simulink model "ur5_simulink_ros2_ibvs_mpc_old"  (R2023b)
settings: Solver=FixedStepAuto  StartTime=0.0  StopTime=inf  RelTol=1e-3
model workspace (MAT data in the model file):
  SL_ROS_VariableLengthArrays_MaxSizes.CommonInfo.ArrayTruncateAction = 'EmitWarning'
  SL_ROS_VariableLengthArrays_MaxSizes.MsgTypeMap = containers.Map
  SL_ROS_VariableLengthArrays_MaxSizes.MsgTypeMap.serialization.keys = {'example_interfaces/Float64MultiArray'}
  SL_ROS_VariableLengthArrays_MaxSizes.MsgTypeMap.serialization.values{1}.PropertyName = 'data'
  SL_ROS_VariableLengthArrays_MaxSizes.MsgTypeMap.serialization.values{1}.DataType = 'double'
  SL_ROS_VariableLengthArrays_MaxSizes.MsgTypeMap.serialization.values{1}.MaxLength = 1
  SL_ROS_VariableLengthArrays_MaxSizes.MsgTypeMap.serialization.uniformity = 0
  SL_ROS_VariableLengthArrays_MaxSizes.MsgTypeMap.serialization.keyType = 'char'
  SL_ROS_VariableLengthArrays_MaxSizes.MsgTypeMap.serialization.valueType = 'any'
undefined symbols (not defined in the file or in its folder): data, data_SL_Info
libraries: ros2lib x12, robotmaniplib x3, robotcorelib x2, mpclib x1, spsFirstOrderFilterLib x1
settings Model: SimulationMode=accelerator  Creator=81232  LastModifiedBy=ias-lab-701
settings OptimizationCC: EnhancedBackFolding=on  PassReuseOutputArgsAs=Individual arguments  ZeroExternalMemoryAtStartup=off  ZeroInternalMemoryAtStartup=off  MaxStackSize=64  OptimizeBlockOrder=speed  DifferentSizesBufferReuse=on  OptimizationCustomize=off  EfficientTunableParamExpr=on
settings DebuggingCC: ParameterTunabilityLossMsg=error
settings ModelReferenceCC: EnableRefExpFcnMdlSchedulingChecks=on
settings SFSimCC: MATLABDynamicMemAlloc=off
settings RTWCC: Description=Embedded Coder  SystemTargetFile=ert.tlc  HardwareBoard=Robot Operating System 2 (ROS 2)  TLCOptions="-aInlineSetEventsForThisBaseRateFcn=TLC_FALSE -aSuppressMultiTaskScheduler=TLC_FALSE  -aRateBasedStepFcn=0"  TemplateMakefile=ert_default_tmf  Toolchain=Colcon Tools  TargetLang=C++
settings CodeAppCC: ForceParamTrailComments=on  IgnoreCustomStorageClasses=off  OperatorAnnotations=on  SimulinkDataObjDesc=on  SFDataObjDesc=on  InsertBlockDesc=on
settings ERTTargetCC: CodeInterfacePackaging=C++ class  RootIOFormat=Structure reference

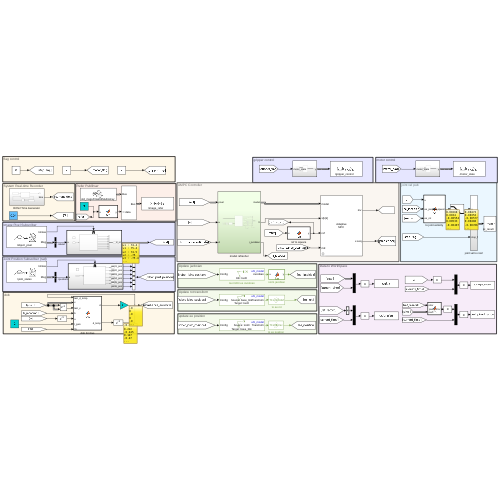
[thumbnail: Simulink's stored preview of the top-level diagram]
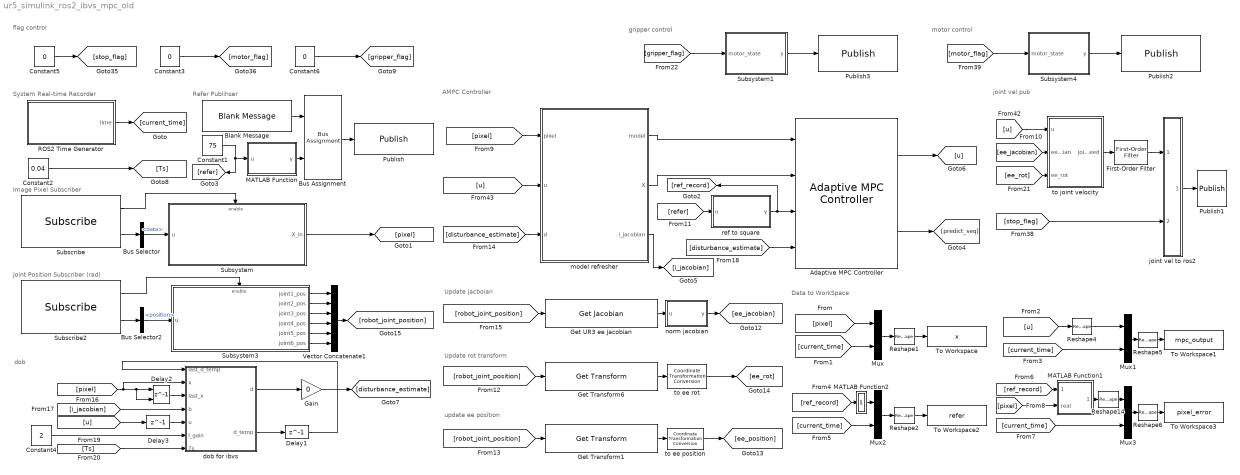
== system ur5_simulink_ros2_ibvs_mpc_old ==
  note: dob
  note: joint vel pub
  note: update ee position
  note: Update rot transform
  note: Joint Position Subscriber (rad)
  note: Refer Publihser
  note: Data to WorkSpace
  note: System Real-time Recorder
  note: Image Pixel Subscriber
  note: AMPC Controller
  note: Update jacboian
  note: flag control
  note: motor control
  note: gripper control
  Adaptive MPC Controller : mpclib/Adaptive MPC Controller  SCDEnableBlockLinearizationSpecification=on  mpcobj=mpcobj  enable_value=0  updateMPCinCallerWorkspace=on  md_inport=on  mv_inport=off  uref_inport=off  return_cost=off  return_mvseq=off  return_qpstatus=off  return_xseq=on  return_state=off  return_ovseq=off  state_inport=on  isltv_plant=off  umin_inport=off  umax_inport=off  ymin_inport=off  ymax_inport=off  cc_inport=off  ywt_inport=off  uwt_inport=off  duwt_inport=off  rhoeps_inport=off  pm_inport=off  MaximumP=10  HorizonChoice=FixedHorizon  BlockDataType=double  SampleTimeInherited=off  switch_inport=off
  Blank Message : ros2lib/Blank Message  messageClass=Message  entityType=std_msgs/Float64MultiArray  messageType=std_msgs/Float64MultiArray  SampleTime=inf
      settings: LibrarySourceBlock=roslib/ROS 2/Blank Message
  Bus Assignment : BusAssignment  AssignedSignals=data
  Bus Selector : BusSelector  OutputSignals=data
  Bus Selector2 : BusSelector  OutputSignals=position
  Constant1 : Constant  Value=75
  Constant2 : Constant  Value=0.04
  Constant3 : Constant  Value=0
  Constant4 : Constant  Value=2
  Constant5 : Constant  Value=0
  Constant6 : Constant  Value=0
  Delay1 : Delay  DelayLength=1
  Delay2 : Delay  DelayLength=1  InitialConditionSource=Input port
      settings: InputPortMap=u0,p4
  Delay3 : Delay  DelayLength=1
  First-Order Filter : spsFirstOrderFilterLib/First-Order Filter  FilterType=Lowpass  Tc=10e-2  Ts=0  Initialize=off  Vac_Init=[0, 0, 60]  Vdc_Init=0  PlotResponse=off  FreqRange="[0,  200,  1]"
  Gain : Gain  Gain=0
  Get Transform1 : robotmaniplib/Get Transform  RigidBodyTree=ur5_model  SourceBody=tool0  TargetBody=base_link  SimulateUsing=Interpreted execution
  Get Transform6 : robotmaniplib/Get Transform  RigidBodyTree=ur5_model  SourceBody=base_link  TargetBody=tool0  SimulateUsing=Interpreted execution
  Get UR3 ee Jacobian : robotmaniplib/Get Jacobian  RigidBodyTree=ur5_model  EndEffector=tool0  SimulateUsing=Interpreted execution
  MATLAB Function : MATLAB Function  TreatAsAtomicUnit=on
  MATLAB Function1 : MATLAB Function  TreatAsAtomicUnit=on
  MATLAB Function2 : MATLAB Function  TreatAsAtomicUnit=on
  Mux{,1..3} (4 alike) : Mux  Inputs=2
  Publish : ros2lib/Publish  topicSource=Specify your own  topic=/image_refer  messageType=std_msgs/Float64MultiArray  QOSHistory=Keep last  QOSDepth=1  QOSReliability=Reliable  QOSDurability=Volatile
      settings: LibrarySourceBlock=roslib/ROS 2/Publish
  Publish1 : ros2lib/Publish  topicSource=Select from ROS network  topic=/simulink_mpc_result  messageType=std_msgs/Float64MultiArray  QOSHistory=Keep last  QOSDepth=1  QOSReliability=Reliable  QOSDurability=Volatile
      settings: LibrarySourceBlock=roslib/ROS 2/Publish
  Publish2 : ros2lib/Publish  topicSource=Select from ROS network  topic=/motor_state  messageType=std_msgs/Int64  QOSHistory=Keep last  QOSDepth=1  QOSReliability=Reliable  QOSDurability=Volatile
      settings: LibrarySourceBlock=roslib/ROS 2/Publish
  Publish3 : ros2lib/Publish  topicSource=Select from ROS network  topic=/gripper_control  messageType=std_msgs/Int64  QOSHistory=Keep last  QOSDepth=1  QOSReliability=Reliable  QOSDurability=Volatile
      settings: LibrarySourceBlock=roslib/ROS 2/Publish
  ROS2 Time Generator : Subsystem
  Reshape1 : Reshape  OutputDimensionality=Customize  OutputDimensions=[9]
  Reshape14 : Reshape  OutputDimensionality=Customize  OutputDimensions=[8,1]
  Reshape2 : Reshape  OutputDimensionality=Customize  OutputDimensions=[9]
  Reshape4 : Reshape  OutputDimensionality=Customize  OutputDimensions=[6,1]
  Reshape5 : Reshape  OutputDimensionality=Customize  OutputDimensions=[7]
  Reshape6 : Reshape  OutputDimensionality=Customize  OutputDimensions=[9]
  Subscribe : ros2lib/Subscribe  topicSource=Select from ROS network  topic=/object_pixel  messageType=std_msgs/Float64MultiArray  sampleTime=-1  QOSHistory=Keep last  QOSDepth=1  QOSReliability=Reliable  QOSDurability=Volatile
  Subscribe2 : ros2lib/Subscribe  topicSource=Select from ROS network  topic=/joint_states  messageType=sensor_msgs/JointState  sampleTime=-1  QOSHistory=Keep last  QOSDepth=1  QOSReliability=Reliable  QOSDurability=Volatile
  Subsystem : Subsystem
  Subsystem1 : Subsystem
  Subsystem3 : Subsystem
  Subsystem4 : Subsystem
  To Workspace : ToWorkspace  VariableName=x  SaveFormat=Timeseries  SampleTime=-1
  To Workspace1 : ToWorkspace  VariableName=mpc_output  SaveFormat=Timeseries  SampleTime=-1
  To Workspace2 : ToWorkspace  VariableName=refer  SaveFormat=Timeseries  SampleTime=-1
  To Workspace3 : ToWorkspace  VariableName=pixel_error  SaveFormat=Timeseries  SampleTime=-1
  Vector Concatenate1 : Concatenate  NumInputs=6
  dob for ibvs : MATLAB Function  TreatAsAtomicUnit=on
  joint vel to ros2 : Subsystem
  model refresher : Subsystem
  norm jacobian : MATLAB Function  TreatAsAtomicUnit=on
  ref to square : MATLAB Function  TreatAsAtomicUnit=on
  to ee position : robotcorelib/Coordinate Transformation Conversion  InputRepresentation=Homogeneous Transformation  InputEulerSequence=ZYX  ShowTrVecInputPort=on  OutputRepresentation=Translation Vector  OutputEulerSequence=ZYX  ShowTrVecOutputPort=off  SimulateUsing=Interpreted execution
  to ee rot : robotcorelib/Coordinate Transformation Conversion  InputRepresentation=Homogeneous Transformation  InputEulerSequence=ZYX  ShowTrVecInputPort=on  OutputRepresentation=Rotation Matrix  OutputEulerSequence=ZYX  ShowTrVecOutputPort=off  SimulateUsing=Interpreted execution
  to joint velocity : MATLAB Function  TreatAsAtomicUnit=on
  wires:
  Bus Selector/1 -> Subsystem/1(u)  "<data>"
  Subscribe/2 -> Bus Selector/1
  Subscribe/1 -> Subsystem/Enable
  ROS2 Time Generator/1(time) -> [current_time]
  Subsystem/1(X_in) -> [pixel]
  [pixel] -> Mux/1
  [current_time] -> Mux/2
  [u] -> Reshape4/1
  [current_time] -> Mux1/2
  Blank Message/1 -> Bus Assignment/1
  Bus Assignment/1 -> Publish/1
  Constant1/1 -> [refer], MATLAB Function/1(u)
  MATLAB Function/1(y) -> Bus Assignment/2
  [current_time] -> Mux2/2
  Mux2/1 -> Reshape2/1
  [current_time] -> Mux3/2
  [ref_record] -> MATLAB Function1/1(refer)
  [pixel] -> MATLAB Function1/2(real)
  ref to square/1(y) -> [ref_record], Adaptive MPC Controller/3
  [refer] -> ref to square/1(u)
  [disturbance_estimate] -> Adaptive MPC Controller/4
  joint vel to ros2/1(Out1) -> Publish1/1
  Adaptive MPC Controller/2 -> [predict_seq]
  Mux3/1 -> Reshape6/1
  MATLAB Function1/1(pixel_error) -> Reshape14/1
  Reshape14/1 -> Mux3/1
  Reshape4/1 -> Mux1/1
  Mux1/1 -> Reshape5/1
  Reshape5/1 -> To Workspace1/1
  Reshape6/1 -> To Workspace3/1
  Subscribe2/2 -> Bus Selector2/1
  Bus Selector2/1 -> Subsystem3/1(u)  "<position>"
  Subscribe2/1 -> Subsystem3/Enable
  model refresher/1(model) -> Adaptive MPC Controller/1
  model refresher/2(X) -> Adaptive MPC Controller/2
  Subsystem3/1(joint1_pos) -> Vector Concatenate1/1
  Subsystem3/2(joint2_pos) -> Vector Concatenate1/2
  Subsystem3/3(joint3_pos) -> Vector Concatenate1/3
  Subsystem3/4(joint4_pos) -> Vector Concatenate1/4
  Subsystem3/5(joint5_pos) -> Vector Concatenate1/5
  Subsystem3/6(joint6_pos) -> Vector Concatenate1/6
  norm jacobian/1(y) -> [ee_jacobian]
  Get UR3 ee Jacobian/1 -> norm jacobian/1(u)
  [pixel] -> model refresher/1(pixel)
  [robot_joint_position] -> Get Transform6/1
  Get Transform6/1 -> to ee rot/1
  to ee rot/1 -> [ee_rot]
  to ee position/1 -> [ee_position]
  Get Transform1/1 -> to ee position/1
  [robot_joint_position] -> Get UR3 ee Jacobian/1
  [robot_joint_position] -> Get Transform1/1
  Vector Concatenate1/1 -> [robot_joint_position]
  [u] -> model refresher/2(u)
  [disturbance_estimate] -> model refresher/3(d)
  Mux/1 -> Reshape1/1
  Reshape1/1 -> To Workspace/1
  Reshape2/1 -> To Workspace2/1
  Delay1/1 -> dob for ibvs/1(last_d_temp)
  [u] -> Delay3/1
  dob for ibvs/2(d_temp) -> Delay1/1
  [i_jacobian] -> dob for ibvs/4(b)
  Constant4/1 -> dob for ibvs/6(l_gain)
  [pixel] -> Delay2/2, Delay2/1, dob for ibvs/2(x)
  Delay2/1 -> dob for ibvs/3(last_x)
  Delay3/1 -> dob for ibvs/5(u)
  Gain/1 -> [disturbance_estimate]
  MATLAB Function2/1(y) -> Mux2/1
  [ref_record] -> MATLAB Function2/1(u)
  dob for ibvs/1(d) -> Gain/1
  [Ts] -> dob for ibvs/7(Ts)
  Constant2/1 -> [Ts]
  Constant5/1 -> [stop_flag]
  Constant3/1 -> [motor_flag]
  [motor_flag] -> Subsystem4/1(motor_state)
  Subsystem4/1(y) -> Publish2/1
  [stop_flag] -> joint vel to ros2/2(stop_flag)
  Constant6/1 -> [gripper_flag]
  Subsystem1/1(y) -> Publish3/1
  [gripper_flag] -> Subsystem1/1(motor_state)
  [u] -> to joint velocity/1(u)
  [ee_jacobian] -> to joint velocity/2(ee_jacobian)
  [ee_rot] -> to joint velocity/3(ee_rot)
  Adaptive MPC Controller/1 -> [u]
  to joint velocity/1(joint_speed) -> First-Order Filter/1
  First-Order Filter/1 -> joint vel to ros2/1(u)
  model refresher/3(i_jacobian) -> [i_jacobian]

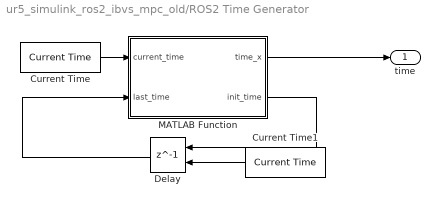
== system ur5_simulink_ros2_ibvs_mpc_old/ROS2 Time Generator ==
  Current Time : ros2lib/Current Time  OutputFormat=double  SampleTime=-1  ModelName=ur5_simulink_ros2_ibvs_mpc_old
      settings: LibrarySourceBlock=roslib/ROS 2/Current Time
  Current Time1 : ros2lib/Current Time  OutputFormat=double  SampleTime=-1  ModelName=ur5_simulink_ros2_ibvs_mpc_old
      settings: LibrarySourceBlock=roslib/ROS 2/Current Time
  Delay : Delay  DelayLength=1  InitialConditionSource=Input port
      settings: InputPortMap=u0,p4
  MATLAB Function : MATLAB Function  TreatAsAtomicUnit=on
  time : Outport
  wires:
  Delay/1 -> MATLAB Function/2(last_time)
  Current Time1/1 -> Delay/2
  MATLAB Function/2(init_time) -> Delay/1
  Current Time/1 -> MATLAB Function/1(current_time)
  MATLAB Function/1(time_x) -> time/1

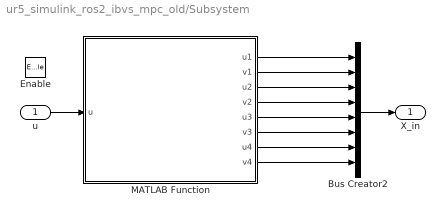
== system ur5_simulink_ros2_ibvs_mpc_old/Subsystem ==
  u : Inport
  Enable : EnablePort
  Bus Creator2 : BusCreator  Inputs=8
  MATLAB Function : MATLAB Function  TreatAsAtomicUnit=on
  X_in : Outport
  wires:
  MATLAB Function/2(v1) -> Bus Creator2/2
  MATLAB Function/5(u3) -> Bus Creator2/5
  MATLAB Function/1(u1) -> Bus Creator2/1
  MATLAB Function/4(v2) -> Bus Creator2/4
  MATLAB Function/3(u2) -> Bus Creator2/3
  u/1 -> MATLAB Function/1(u)
  Bus Creator2/1 -> X_in/1
  MATLAB Function/6(v3) -> Bus Creator2/6
  MATLAB Function/7(u4) -> Bus Creator2/7
  MATLAB Function/8(v4) -> Bus Creator2/8

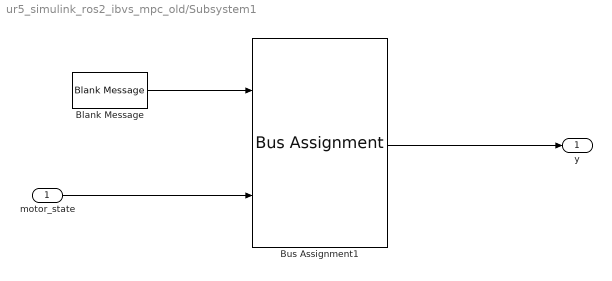
== system ur5_simulink_ros2_ibvs_mpc_old/Subsystem1 ==
  motor_state : Inport
  Blank Message : ros2lib/Blank Message  messageClass=Message  entityType=std_msgs/Int64  messageType=std_msgs/Int64  SampleTime=inf
  Bus Assignment1 : BusAssignment  AssignedSignals=data
  y : Outport
  wires:
  Blank Message/1 -> Bus Assignment1/1
  Bus Assignment1/1 -> y/1
  motor_state/1 -> Bus Assignment1/2

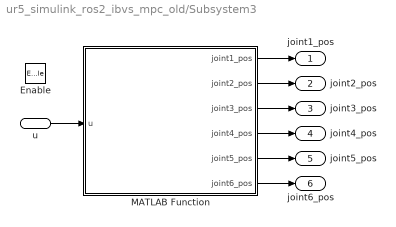
== system ur5_simulink_ros2_ibvs_mpc_old/Subsystem3 ==
  u : Inport
  Enable : EnablePort
  MATLAB Function : MATLAB Function  TreatAsAtomicUnit=on
  joint1_pos : Outport
  joint2_pos : Outport  Port=2
  joint3_pos : Outport  Port=3
  joint4_pos : Outport  Port=4
  joint5_pos : Outport  Port=5
  joint6_pos : Outport  Port=6
  wires:
  u/1 -> MATLAB Function/1(u)
  MATLAB Function/1(joint1_pos) -> joint1_pos/1
  MATLAB Function/2(joint2_pos) -> joint2_pos/1
  MATLAB Function/3(joint3_pos) -> joint3_pos/1
  MATLAB Function/4(joint4_pos) -> joint4_pos/1
  MATLAB Function/5(joint5_pos) -> joint5_pos/1
  MATLAB Function/6(joint6_pos) -> joint6_pos/1

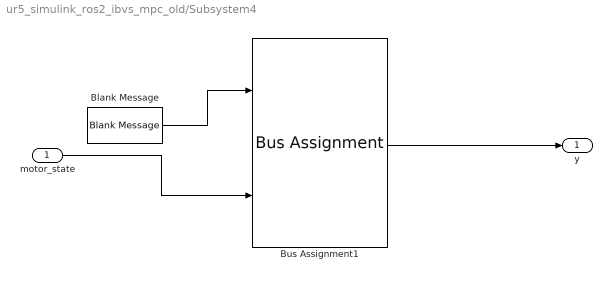
== system ur5_simulink_ros2_ibvs_mpc_old/Subsystem4 ==
  motor_state : Inport
  Blank Message : ros2lib/Blank Message  messageClass=Message  entityType=std_msgs/Int64  messageType=std_msgs/Int64  SampleTime=inf
  Bus Assignment1 : BusAssignment  AssignedSignals=data
  y : Outport
  wires:
  Blank Message/1 -> Bus Assignment1/1
  Bus Assignment1/1 -> y/1
  motor_state/1 -> Bus Assignment1/2

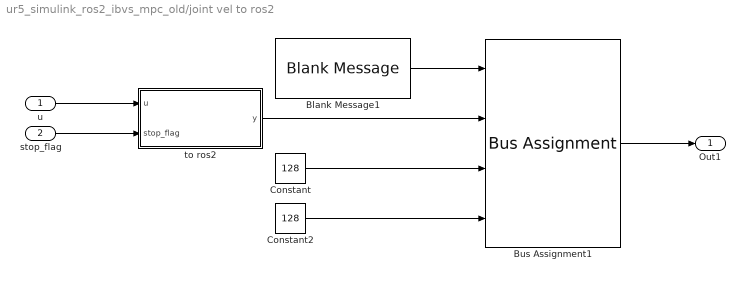
== system ur5_simulink_ros2_ibvs_mpc_old/joint vel to ros2 ==
  u : Inport
  stop_flag : Inport  Port=2
  Blank Message1 : ros2lib/Blank Message  messageClass=Message  entityType=std_msgs/Float64MultiArray  messageType=std_msgs/Float64MultiArray  SampleTime=inf
      settings: LibrarySourceBlock=roslib/ROS 2/Blank Message
  Bus Assignment1 : BusAssignment  AssignedSignals=data,data_SL_Info.CurrentLength,data_SL_Info.ReceivedLength
  Constant : Constant  Value=128  OutDataTypeStr=uint32
  Constant2 : Constant  Value=128  OutDataTypeStr=uint32
  to ros2 : MATLAB Function  TreatAsAtomicUnit=on
  Out1 : Outport
  wires:
  u/1 -> to ros2/1(u)
  to ros2/1(y) -> Bus Assignment1/2
  Constant2/1 -> Bus Assignment1/4
  Constant/1 -> Bus Assignment1/3
  Blank Message1/1 -> Bus Assignment1/1
  Bus Assignment1/1 -> Out1/1
  stop_flag/1 -> to ros2/2(stop_flag)

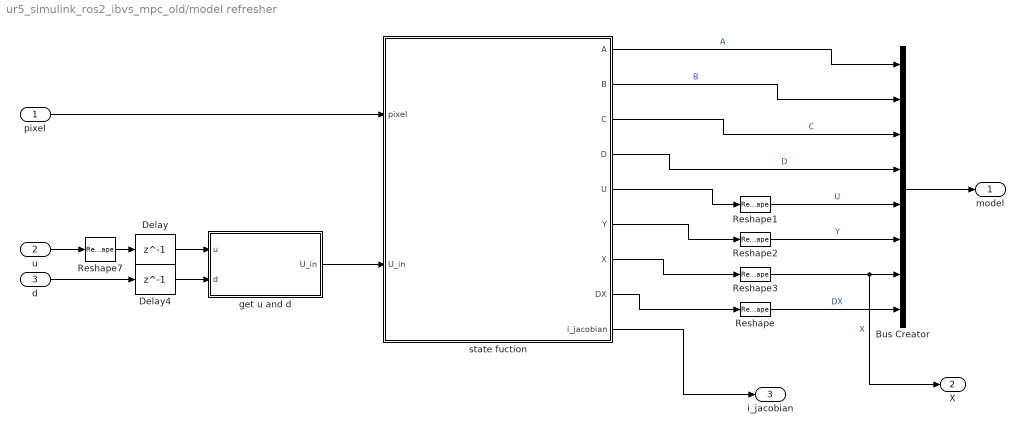
== system ur5_simulink_ros2_ibvs_mpc_old/model refresher ==
  pixel : Inport
  u : Inport  Port=2
  d : Inport  Port=3
  Bus Creator : BusCreator  Inputs=8
  Delay : Delay  DelayLength=1
  Delay4 : Delay  DelayLength=1
  Reshape : Reshape  OutputDimensionality=Customize  OutputDimensions=[8,1]
  Reshape1 : Reshape  OutputDimensionality=Customize  OutputDimensions=[14,1]
  Reshape2 : Reshape  OutputDimensionality=Customize  OutputDimensions=[8,1]
  Reshape3 : Reshape  OutputDimensionality=Customize  OutputDimensions=[8,1]
  Reshape7 : Reshape  OutputDimensionality=Customize  OutputDimensions=[6]
  get u and d : Subsystem
  state fuction : MATLAB Function  TreatAsAtomicUnit=on
  model : Outport
  X : Outport  Port=2
  i_jacobian : Outport  Port=3
  wires:
  state fuction/2(B) -> Bus Creator/2  "B"
  state fuction/5(U) -> Reshape1/1
  pixel/1 -> state fuction/1(pixel)
  state fuction/1(A) -> Bus Creator/1  "A"
  state fuction/4(D) -> Bus Creator/4  "D"
  state fuction/3(C) -> Bus Creator/3  "C"
  get u and d/1(U_in) -> state fuction/2(U_in)
  state fuction/6(Y) -> Reshape2/1
  state fuction/7(X) -> Reshape3/1
  state fuction/8(DX) -> Reshape/1
  Reshape1/1 -> Bus Creator/5  "U"
  Reshape2/1 -> Bus Creator/6  "Y"
  Reshape3/1 -> Bus Creator/7, X/1  "X"
  Reshape/1 -> Bus Creator/8  "DX"
  Bus Creator/1 -> model/1
  Reshape7/1 -> Delay/1
  Delay4/1 -> get u and d/2(d)
  Delay/1 -> get u and d/1(u)
  u/1 -> Reshape7/1
  d/1 -> Delay4/1
  state fuction/9(i_jacobian) -> i_jacobian/1

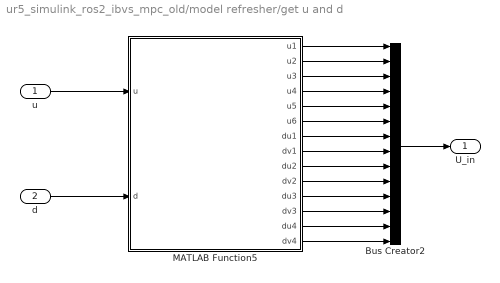
== system ur5_simulink_ros2_ibvs_mpc_old/model refresher/get u and d ==
  u : Inport
  d : Inport  Port=2
  Bus Creator2 : BusCreator  Inputs=14
  MATLAB Function5 : MATLAB Function  TreatAsAtomicUnit=on
  U_in : Outport
  wires:
  MATLAB Function5/3(u3) -> Bus Creator2/3
  MATLAB Function5/1(u1) -> Bus Creator2/1
  MATLAB Function5/11(du3) -> Bus Creator2/11
  MATLAB Function5/8(dv1) -> Bus Creator2/8
  MATLAB Function5/12(dv3) -> Bus Creator2/12
  MATLAB Function5/9(du2) -> Bus Creator2/9
  MATLAB Function5/13(du4) -> Bus Creator2/13
  MATLAB Function5/14(dv4) -> Bus Creator2/14
  MATLAB Function5/6(u6) -> Bus Creator2/6
  MATLAB Function5/4(u4) -> Bus Creator2/4
  MATLAB Function5/5(u5) -> Bus Creator2/5
  MATLAB Function5/7(du1) -> Bus Creator2/7
  MATLAB Function5/2(u2) -> Bus Creator2/2
  MATLAB Function5/10(dv2) -> Bus Creator2/10
  u/1 -> MATLAB Function5/1(u)
  Bus Creator2/1 -> U_in/1
  d/1 -> MATLAB Function5/2(d)

== matlab function ur5_simulink_ros2_ibvs_mpc_old/joint vel to ros2/to ros2 ==
  data: u input; y output; stop_flag input
function y  = fcn(u, stop_flag)
    y = zeros(128,1);
    if stop_flag==1
        y(1) = 0;
        y(2) = 0;
        y(3) = 0;
        y(4) = 0;
        y(5) = 0;
        y(6) = 0;
    else
        y(1) = u(1);
        y(2) = u(2);
        y(3) = u(3);
        y(4) = u(4);
        y(5) = u(5);
        y(6) = u(6);
    end
end

== matlab function ur5_simulink_ros2_ibvs_mpc_old/MATLAB Function2 ==
  data: u input; y output
function y = fcn(u)
y = u(1:8);

== matlab function ur5_simulink_ros2_ibvs_mpc_old/model refresher/get u and d/MATLAB Function5 ==
  data: u input; u1 output; u2 output; u3 output; u4 output; u5 output; u6 output; du1 output; dv1 output; du2 output; dv2 output; du3 output; dv3 output; du4 output; dv4 output; d input
function [u1,u2,u3,u4,u5,u6,du1,dv1,du2,dv2,du3,dv3,du4,dv4] = fcn(u,d)
u1 = u(1);
u2 = u(2);
u3 = u(3);
u4 = u(4);
u5 = u(5);
u6 = u(6);
%disturbance
du1 = d(1);
dv1 = d(2);
du2 = d(3);
dv2 = d(4);
du3 = d(5);
dv3 = d(6);
du4 = d(7);
dv4 = d(8);

== matlab function ur5_simulink_ros2_ibvs_mpc_old/to joint velocity ==
  data: u input; joint_speed output; ee_jacobian input; ee_rot input
function joint_speed  = fcn(u, ee_jacobian, ee_rot)
    rot_mat = [ee_rot,zeros(3,3);zeros(3,3),ee_rot];
    new_jacobian = rot_mat*ee_jacobian;
    joint_speed = new_jacobian\u;
end

== matlab function ur5_simulink_ros2_ibvs_mpc_old/norm jacobian ==
  data: u input; y output size=[6,6]
function y = fcn(u)
firstThreeColumns =u(1:3, :);
lastThreeColumns = u(4:6, :);
y = [lastThreeColumns;firstThreeColumns];

== matlab function ur5_simulink_ros2_ibvs_mpc_old/Subsystem3/MATLAB Function ==
  data: u input; joint1_pos output; joint2_pos output; joint3_pos output; joint4_pos output; joint5_pos output; joint6_pos output
function [joint1_pos,joint2_pos,joint3_pos,joint4_pos,joint5_pos,joint6_pos] = fcn(u)
joint1_pos = u(6);
joint2_pos = u(1);
joint3_pos = u(2);
joint4_pos = u(3);
joint5_pos = u(4);
joint6_pos = u(5);

== matlab function ur5_simulink_ros2_ibvs_mpc_old/Subsystem/MATLAB Function ==
  data: u input; u1 output; v1 output; u2 output; v2 output; u3 output; v3 output; u4 output; v4 output
function [u1,v1,u2,v2,u3,v3,u4,v4] = fcn(u)
u_center = 320;
v_center = 240;
u1 = u(1) - u_center;
v1 = u(2) - v_center;
u2 = u(3) - u_center;
v2 = u(4) - v_center;
u3 = u(5) - u_center;
v3 = u(6) - v_center;
u4 = u(7) - u_center;
v4 = u(8) - v_center;

== matlab function ur5_simulink_ros2_ibvs_mpc_old/ROS2 Time Generator/MATLAB Function ==
  data: current_time input; last_time input; time_x output; init_time output
function [time_x,init_time] = fcn(current_time, last_time)
init_time = last_time;
time_x = current_time-last_time;

== matlab function ur5_simulink_ros2_ibvs_mpc_old/dob for ibvs ==
  data: last_d_temp input size=8; x input size=8; last_x input size=8; b input size=[8,6]; u input size=6; d output size=8; l_gain input; d_temp output size=8; Ts input
function [d,d_temp] = fcn(last_d_temp,x,last_x,b,u,l_gain,Ts)
d_temp = last_d_temp - Ts*l_gain*last_d_temp + l_gain*(x-last_x-Ts*b*u);
d = d_temp;

== matlab function ur5_simulink_ros2_ibvs_mpc_old/MATLAB Function ==
  data: u input; y output
function y = fcn(u)
y = zeros(1,128);
y(1) = u;
y(2) = u;
y(3) = u;
y(4) = -u;
y(5) = -u;
y(6) = -u;
y(7) = -u;
y(8) = u;

== matlab function ur5_simulink_ros2_ibvs_mpc_old/MATLAB Function1 ==
  data: refer input; pixel_error output; real input
function pixel_error = fcn(refer,real)
pixel_error = zeros(8,1);
pixel_error(1) = refer(1) -real(1);
pixel_error(2) = refer(2) -real(2);
pixel_error(3) = refer(3) -real(3);
pixel_error(4) = refer(4) -real(4);
pixel_error(5) = refer(5) -real(5);
pixel_error(6) = refer(6) -real(6);
pixel_error(7) = refer(7) -real(7);
pixel_error(8) = refer(8) -real(8);

== matlab function ur5_simulink_ros2_ibvs_mpc_old/model refresher/state fuction ==
  data: pixel input; A output; U_in input; B output; C output; D output; U output; Y output; X output; DX output; i_jacobian output
function [A, B, C, D, U, Y, X, DX,i_jacobian] = fcn(pixel, U_in)
A = zeros(8,8);
C = eye(8);
D = zeros(8,14);
X= pixel;
[B,i_jacobian] = getContinuous(X);
U=U_in;
DZ = B*U_in;
DX = [DZ(1);DZ(2);DZ(3);DZ(4);DZ(5);DZ(6);DZ(7);DZ(8)];
Y=X;

function  [b_,i_jacobian_] = getContinuous(x_)
b_ = zeros(8, 14);
% states
u_1 = x_(1);
v_1 = x_(2);
u_2 = x_(3);
v_2 = x_(4);
u_3 = x_(5);
v_3 = x_(6);
u_4 = x_(7);
v_4 = x_(8);
% parameters
f = 900;            %focal length of realsenseD455=1930um
p_size = 0;        %Pixel Size of realsenseD4455=3um
f_pixel = 633;       %the focal length in pixels f/p_size
Z = 0.25;             %Depth estimate for four points
% image jcobian
i_jacobian_ = [-f_pixel/Z,0,u_1/Z,u_1*v_1/f_pixel,-(f_pixel^2+u_1^2)/f_pixel,v_1;
             0,-f_pixel/Z,v_1/Z,(f_pixel^2+v_1^2)/f_pixel,-u_1*v_1/f_pixel,-u_1;
             -f_pixel/Z,0,u_2/Z,u_2*v_2/f_pixel,-(f_pixel^2+u_2^2)/f_pixel,v_2;
             0,-f_pixel/Z,v_2/Z,(f_pixel^2+v_2^2)/f_pixel,-u_2*v_2/f_pixel,-u_2;
             -f_pixel/Z,0,u_3/Z,u_3*v_3/f_pixel,-(f_pixel^2+u_3^2)/f_pixel,v_3;
             0,-f_pixel/Z,v_3/Z,(f_pixel^2+v_3^2)/f_pixel,-u_3*v_3/f_pixel,-u_3;
             -f_pixel/Z,0,u_4/Z,u_4*v_4/f_pixel,-(f_pixel^2+u_4^2)/f_pixel,v_4;
             0,-f_pixel/Z,v_4/Z,(f_pixel^2+v_4^2)/f_pixel,-u_4*v_4/f_pixel,-u_4];
disturbance_mat = eye(8);

% state equations
b_(1:8, 1:6) = i_jacobian_;
b_(1:8, 7:14) = disturbance_mat;

== matlab function ur5_simulink_ros2_ibvs_mpc_old/ref to square ==
  data: u input; y output size=[8,1]
function y = fcn(u)
y = zeros(8,1);
y(1) = u;
y(2) = u;
y(3) = u;
y(4) = -u;
y(5) = -u;
y(6) = -u;
y(7) = -u;
y(8) = u;
